simulink model "kurtosis_single_channel_subblocks"  (R2012b)
settings: Solver=ode45  StartTime=0.0  StopTime=3571  RelTol=1e-3
libraries: xbsIndex_r4 x454, xps_library x2, simulink_xsg_bridge x1
(part 2 of 4)

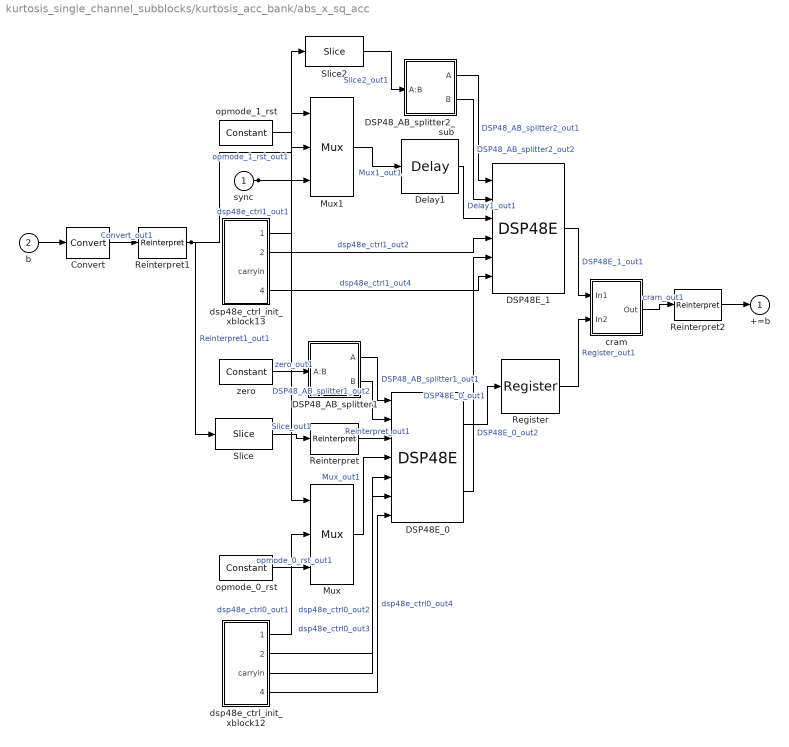
== system kurtosis_single_channel_subblocks/kurtosis_acc_bank/abs_x_sq_acc ==
  sync : Inport
  b : Inport  Port=2
  Convert : xbsIndex_r4/Convert  gui_display_data_type=Fixed-point  arith_type="Signed  (2's comp)"  n_bits=96  bin_pt=34  float_type=Single  exp_bits=8  fraction_bits=24  quantization=Truncate  overflow=Wrap  en=off  latency=0  dbl_ovrd=off  pipeline=off  block_type=convert
  DSP48E_0 : xbsIndex_r4/DSP48E  use_a=Direct from A Port  use_b=Direct from B Port  reset_preg=off  pattern_from_creg=on  pattern='000000000000'  mask_from_creg=on  pattern_mask='000000000000'  sel_rounding_mask=Select mask  use_op=off  use_creg=on  rst_all=off  en_all=off  use_pcin=off  use_carrycascin=off  use_multsignin=off  use_carryout=on  use_patterndetect=off  use_patternbdetect=off  use_overflow=off  use_underflow=off  use_acout=off  use_bcout=off  use_pcout=off  use_multsignout=off  use_carrycascout=off  pipeline_a=1  pipeline_b=1  pipeline_acout=1  pipeline_bcout=1  pipeline_c=on  pipeline_p=on  pipeline_mult=on  pipeline_opmode=on  pipeline_alumode=on  pipeline_carryin=on  pipeline_carryinsel=on  rst_a=off  rst_b=off  rst_c=off  rst_mult=off  rst_p=off  rst_carry_in=off  rst_alumode=off  rst_ctrl=off  en_a1=off  en_a2=off  en_b1=off  en_b2=off  en_c=off  en_mult=off  en_p=off  en_carry_in=off  en_alumode=off  en_multcarryin=off  en_ctrl=off  use_synth_model=off  addsub_mode=ONE48  xl_useadderonly=off  block_type=dsp48e
  DSP48E_1 : xbsIndex_r4/DSP48E  use_a=Direct from A Port  use_b=Direct from B Port  reset_preg=off  pattern_from_creg=on  pattern='000000000000'  mask_from_creg=on  pattern_mask='000000000000'  sel_rounding_mask=Select mask  use_op=off  use_creg=off  rst_all=off  en_all=off  use_pcin=off  use_carrycascin=off  use_multsignin=off  use_carryout=off  use_patterndetect=off  use_patternbdetect=off  use_overflow=off  use_underflow=off  use_acout=off  use_bcout=off  use_pcout=off  use_multsignout=off  use_carrycascout=off  pipeline_a=2  pipeline_b=2  pipeline_acout=1  pipeline_bcout=1  pipeline_c=on  pipeline_p=on  pipeline_mult=on  pipeline_opmode=on  pipeline_alumode=on  pipeline_carryin=off  pipeline_carryinsel=on  rst_a=off  rst_b=off  rst_c=off  rst_mult=off  rst_p=off  rst_carry_in=off  rst_alumode=off  rst_ctrl=off  en_a1=off  en_a2=off  en_b1=off  en_b2=off  en_c=off  en_mult=off  en_p=off  en_carry_in=off  en_alumode=off  en_multcarryin=off  en_ctrl=off  use_synth_model=off  addsub_mode=ONE48  xl_useadderonly=off  block_type=dsp48e
  DSP48_AB_splitter1 : Subsystem
  DSP48_AB_splitter2_sub : Subsystem
  Delay1 : xbsIndex_r4/Delay  rst=off  infoeditControl=Selection of Reset will increase slice count due to use of real FFs and instead of SRLs  en=off  latency=1  dbl_ovrd=off  reg_retiming=off  block_type=delay
  Mux : xbsIndex_r4/Mux  inputs=2  en=off  latency=0  precision=Full  arith_type=Unsigned  n_bits=16  bin_pt=14  quantization=Truncate  overflow=Wrap  dbl_ovrd=off  block_type=mux
  Mux1 : xbsIndex_r4/Mux  inputs=2  en=off  latency=0  precision=Full  arith_type=Unsigned  n_bits=16  bin_pt=14  quantization=Truncate  overflow=Wrap  dbl_ovrd=off  block_type=mux
  Register : xbsIndex_r4/Register  init=0  rst=off  en=off  dbl_ovrd=off  block_type=register
  Reinterpret : xbsIndex_r4/Reinterpret  force_arith_type=on  arith_type="Signed  (2's comp)"  force_bin_pt=on  bin_pt=0  block_type=reinterpret
  Reinterpret1 : xbsIndex_r4/Reinterpret  force_arith_type=on  arith_type="Signed  (2's comp)"  force_bin_pt=on  bin_pt=0  block_type=reinterpret
  Reinterpret2 : xbsIndex_r4/Reinterpret  force_arith_type=on  arith_type="Signed  (2's comp)"  force_bin_pt=on  bin_pt=34  block_type=reinterpret
  Slice : xbsIndex_r4/Slice  nbits=48  boolean_output=off  mode=Lower Bit Location + Width  bit1=0  base1=MSB of Input  bit0=0  base0=LSB of Input  dbl_ovrd=off  block_type=slice
  Slice2 : xbsIndex_r4/Slice  nbits=48  boolean_output=off  mode=Lower Bit Location + Width  bit1=0  base1=MSB of Input  bit0=48  base0=LSB of Input  dbl_ovrd=off  block_type=slice
  cram : Subsystem
  dsp48e_ctrl_init_xblock12 : Subsystem
  dsp48e_ctrl_init_xblock13 : Subsystem
  opmode_0_rst : xbsIndex_r4/Constant  const=12  gui_display_data_type=Fixed-point  arith_type=Unsigned  n_bits=7  bin_pt=0  preci_type=Single  exp_width=8  frac_width=24  explicit_period=on  period=1  equ=P=C  opselect=C  inp2=PCIN>>17  opr=+  inp1=P  carry=CIN  dbl_ovrd=off  block_type=constant
  opmode_1_rst : xbsIndex_r4/Constant  const=3  gui_display_data_type=Fixed-point  arith_type=Unsigned  n_bits=7  bin_pt=0  preci_type=Single  exp_width=8  frac_width=24  explicit_period=on  period=1  equ=P=C  opselect=C  inp2=PCIN>>17  opr=+  inp1=P  carry=CIN  dbl_ovrd=off  block_type=constant
  zero : xbsIndex_r4/Constant  const=0  gui_display_data_type=Fixed-point  arith_type=Signed (2's comp)  n_bits=48  bin_pt=0  preci_type=Single  exp_width=8  frac_width=24  explicit_period=on  period=1  equ=P=C  opselect=C  inp2=PCIN>>17  opr=+  inp1=P  carry=CIN  dbl_ovrd=off  block_type=constant
  +=b : Outport
  wires:
  sync/1 -> Mux1/1, Mux/1
  Reinterpret1/1 -> Slice2/1, Slice/1  "Reinterpret1_out1"
  dsp48e_ctrl_init_xblock13/4(carryinsel) -> DSP48E_1/6  "dsp48e_ctrl1_out4"
  dsp48e_ctrl_init_xblock13/2(alumode) -> DSP48E_1/4  "dsp48e_ctrl1_out2"
  dsp48e_ctrl_init_xblock13/1(opmode) -> Mux1/2  "dsp48e_ctrl1_out1"
  dsp48e_ctrl_init_xblock12/4(carryinsel) -> DSP48E_0/7  "dsp48e_ctrl0_out4"
  dsp48e_ctrl_init_xblock12/3(carryin) -> DSP48E_0/6  "dsp48e_ctrl0_out3"
  dsp48e_ctrl_init_xblock12/2(alumode) -> DSP48E_0/5  "dsp48e_ctrl0_out2"
  dsp48e_ctrl_init_xblock12/1(opmode) -> Mux/2  "dsp48e_ctrl0_out1"
  DSP48_AB_splitter2_sub/2(B) -> DSP48E_1/2  "DSP48_AB_splitter2_out2"
  DSP48_AB_splitter2_sub/1(A) -> DSP48E_1/1  "DSP48_AB_splitter2_out1"
  Slice2/1 -> DSP48_AB_splitter2_sub/1(A:B)  "Slice2_out1"
  zero/1 -> DSP48_AB_splitter1/1(A:B)  "zero_out1"
  opmode_1_rst/1 -> Mux1/3  "opmode_1_rst_out1"
  opmode_0_rst/1 -> Mux/3  "opmode_0_rst_out1"
  cram/1(Out) -> Reinterpret2/1  "cram_out1"
  Register/1 -> cram/2(In2)  "Register_out1"
  DSP48E_1/1 -> cram/1(In1)  "DSP48E_1_out1"
  Slice/1 -> Reinterpret/1  "Slice_out1"
  Reinterpret2/1 -> +=b/1
  Convert/1 -> Reinterpret1/1  "Convert_out1"
  Reinterpret/1 -> DSP48E_0/3  "Reinterpret_out1"
  DSP48E_0/1 -> Register/1  "DSP48E_0_out1"
  Mux1/1 -> Delay1/1  "Mux1_out1"
  Mux/1 -> DSP48E_0/4  "Mux_out1"
  Delay1/1 -> DSP48E_1/3  "Delay1_out1"
  DSP48_AB_splitter1/2(B) -> DSP48E_0/2  "DSP48_AB_splitter1_out2"
  DSP48_AB_splitter1/1(A) -> DSP48E_0/1  "DSP48_AB_splitter1_out1"
  DSP48E_0/2 -> DSP48E_1/5  "DSP48E_0_out2"
  b/1 -> Convert/1

== system kurtosis_single_channel_subblocks/kurtosis_acc_bank/acc_rst ==
  sync : Inport
  Constant5 : xbsIndex_r4/Constant  const=1023  gui_display_data_type=Fixed-point  arith_type=Unsigned  n_bits=11  bin_pt=0  preci_type=Single  exp_width=8  frac_width=24  explicit_period=on  period=1  equ=P=C  opselect=C  inp2=PCIN>>17  opr=+  inp1=P  carry=CIN  dbl_ovrd=off  block_type=constant
  Counter : xbsIndex_r4/Counter  cnt_type=Free Running  cnt_to=Inf  operation=Up  start_count=0  cnt_by_val=1  arith_type=Unsigned  n_bits=10  bin_pt=0  load_pin=off  rst=on  en=off  explicit_period=on  period=1  dbl_ovrd=off  use_behavioral_HDL=off  implementation=Fabric  block_type=counter
  Logical : xbsIndex_r4/Logical  logical_function=OR  inputs=2  en=off  latency=0  precision=Full  arith_type=Unsigned  n_bits=16  bin_pt=0  align_bp=on  dbl_ovrd=off  block_type=logical
  Relational : xbsIndex_r4/Relational  mode=a=b  en=off  latency=0  dbl_ovrd=off  block_type=relational
  acc_del : xbsIndex_r4/Delay  rst=off  infoeditControl=Selection of Reset will increase slice count due to use of real FFs and instead of SRLs  en=off  latency=2  dbl_ovrd=off  reg_retiming=off  block_type=delay
  sync_del : xbsIndex_r4/Delay  rst=off  infoeditControl=Selection of Reset will increase slice count due to use of real FFs and instead of SRLs  en=off  latency=1  dbl_ovrd=off  reg_retiming=off  block_type=delay
  acc_rst : Outport
  sync_out : Outport  Port=2
  wires:
  sync/1 -> Logical/2, Counter/1
  Relational/1 -> sync_del/1, acc_del/1  "Relational_out1"
  sync_del/1 -> Logical/1  "sync_del_out1"
  acc_del/1 -> sync_out/1
  Constant5/1 -> Relational/2  "Constant5_out1"
  Counter/1 -> Relational/1  "Counter_out1"
  Logical/1 -> acc_rst/1

== system kurtosis_single_channel_subblocks/kurtosis_acc_bank/x_acc ==
  sync : Inport
  x : Inport  Port=2
  c_to_ri : Subsystem
      settings: AttributesFormatString=55_51 r/i
  im_acc : Subsystem
  re_acc : Subsystem
  x_re_acc : Outport
  x_im_acc : Outport  Port=2
  wires:
  sync/1 -> im_acc/1(sync), re_acc/1(sync)
  im_acc/1(+=b) -> x_im_acc/1
  c_to_ri/2(im) -> im_acc/2(b)  "x_im"
  re_acc/1(+=b) -> x_re_acc/1
  c_to_ri/1(re) -> re_acc/2(b)  "x_re"
  x/1 -> c_to_ri/1(c)

== system kurtosis_single_channel_subblocks/kurtosis_acc_bank/x_cube_acc ==
  sync : Inport
  x : Inport  Port=2
  c_to_ri : Subsystem
  im_acc : Subsystem
  re_acc : Subsystem
  x_re_acc : Outport
  x_im_acc : Outport  Port=2
  wires:
  sync/1 -> im_acc/1(sync), re_acc/1(sync)
  im_acc/1(+=b) -> x_im_acc/1
  c_to_ri/2(im) -> im_acc/2(b)  "x_im"
  re_acc/1(+=b) -> x_re_acc/1
  c_to_ri/1(re) -> re_acc/2(b)  "x_re"
  x/1 -> c_to_ri/1(c)

== system kurtosis_single_channel_subblocks/kurtosis_acc_bank/x_sq_acc ==
  sync : Inport
  x : Inport  Port=2
  c_to_ri : Subsystem
  im_acc : Subsystem
  re_acc : Subsystem
  x_re_acc : Outport
  x_im_acc : Outport  Port=2
  wires:
  sync/1 -> im_acc/1(sync), re_acc/1(sync)
  im_acc/1(+=b) -> x_im_acc/1
  c_to_ri/2(im) -> im_acc/2(b)  "x_im"
  re_acc/1(+=b) -> x_re_acc/1
  c_to_ri/1(re) -> re_acc/2(b)  "x_re"
  x/1 -> c_to_ri/1(c)

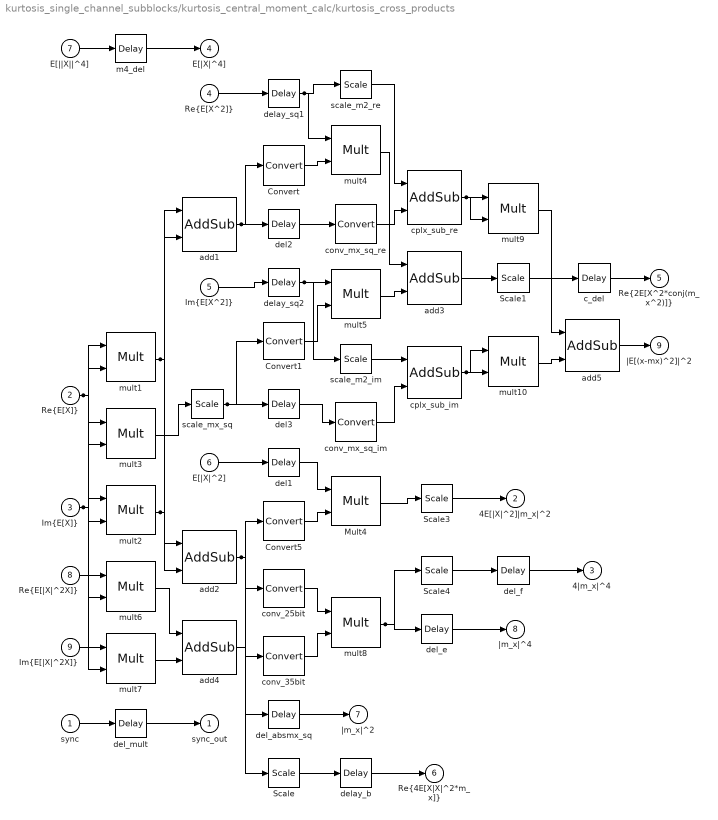
== system kurtosis_single_channel_subblocks/kurtosis_central_moment_calc/kurtosis_cross_products ==
  sync : Inport
  "Re{E[X]}" : Inport  Port=2
  "Im{E[X]}" : Inport  Port=3
  "Re{E[X^2]}" : Inport  Port=4
  "Im{E[X^2]}" : Inport  Port=5
  E[|X|^2] : Inport  Port=6
  E[||X||^4] : Inport  Port=7
  "Re{E[|X|^2X]}" : Inport  Port=8
  "Im{E[|X|^2X]}" : Inport  Port=9
  Convert : xbsIndex_r4/Convert  gui_display_data_type=Fixed-point  arith_type="Signed  (2's comp)"  n_bits=25  bin_pt=22  float_type=Single  exp_bits=8  fraction_bits=24  quantization="Round  (unbiased: +/- Inf)"  overflow=Saturate  en=off  latency=1  dbl_ovrd=off  pipeline=off  block_type=convert
  Convert1 : xbsIndex_r4/Convert  gui_display_data_type=Fixed-point  arith_type="Signed  (2's comp)"  n_bits=25  bin_pt=22  float_type=Single  exp_bits=8  fraction_bits=24  quantization="Round  (unbiased: +/- Inf)"  overflow=Saturate  en=off  latency=1  dbl_ovrd=off  pipeline=off  block_type=convert
  Convert5 : xbsIndex_r4/Convert  gui_display_data_type=Fixed-point  arith_type="Signed  (2's comp)"  n_bits=25  bin_pt=22  float_type=Single  exp_bits=8  fraction_bits=24  quantization="Round  (unbiased: +/- Inf)"  overflow=Saturate  en=off  latency=5  dbl_ovrd=off  pipeline=off  block_type=convert
  Mult4 : xbsIndex_r4/Mult  precision=Full  arith_type="Signed  (2's comp)"  n_bits=36  bin_pt=34  quantization=Truncate  overflow=Wrap  en=off  latency=5  dbl_ovrd=off  use_behavioral_HDL=off  opt=Speed  use_embedded=on  optimum_pipeline=off  pipeline=on  use_rpm=on  placement_style=Triangular  block_type=mult
  Scale : xbsIndex_r4/Scale  scale_factor=2  dbl_ovrd=off  block_type=scale
  Scale1 : xbsIndex_r4/Scale  scale_factor=1  dbl_ovrd=off  block_type=scale
  Scale3 : xbsIndex_r4/Scale  scale_factor=2  dbl_ovrd=off  block_type=scale
  Scale4 : xbsIndex_r4/Scale  scale_factor=2  dbl_ovrd=off  block_type=scale
  add1 : xbsIndex_r4/AddSub  mode=Subtraction  use_carryin=off  use_carryout=off  en=off  latency=2  precision=Full  arith_type="Signed  (2's comp)"  n_bits=36  bin_pt=34  quantization=Truncate  overflow=Wrap  dbl_ovrd=off  use_behavioral_HDL=off  hw_selection=Fabric  pipelined=off  block_type=addsub
  add2 : xbsIndex_r4/AddSub  mode=Addition  use_carryin=off  use_carryout=off  en=off  latency=2  precision=Full  arith_type="Signed  (2's comp)"  n_bits=36  bin_pt=34  quantization=Truncate  overflow=Wrap  dbl_ovrd=off  use_behavioral_HDL=off  hw_selection=Fabric  pipelined=off  block_type=addsub
  add3 : xbsIndex_r4/AddSub  mode=Addition  use_carryin=off  use_carryout=off  en=off  latency=2  precision=Full  arith_type="Signed  (2's comp)"  n_bits=36  bin_pt=34  quantization=Truncate  overflow=Wrap  dbl_ovrd=off  use_behavioral_HDL=off  hw_selection=Fabric  pipelined=off  block_type=addsub
  add4 : xbsIndex_r4/AddSub  mode=Addition  use_carryin=off  use_carryout=off  en=off  latency=2  precision=Full  arith_type="Signed  (2's comp)"  n_bits=36  bin_pt=34  quantization=Truncate  overflow=Wrap  dbl_ovrd=off  use_behavioral_HDL=off  hw_selection=Fabric  pipelined=off  block_type=addsub
  add5 : xbsIndex_r4/AddSub  mode=Addition  use_carryin=off  use_carryout=off  en=off  latency=3  precision=Full  arith_type="Signed  (2's comp)"  n_bits=36  bin_pt=34  quantization=Truncate  overflow=Wrap  dbl_ovrd=off  use_behavioral_HDL=off  hw_selection=Fabric  pipelined=off  block_type=addsub
  c_del : xbsIndex_r4/Delay  rst=off  infoeditControl=Selection of Reset will increase slice count due to use of real FFs and instead of SRLs  en=off  latency=4  dbl_ovrd=off  reg_retiming=off  block_type=delay
  conv_25bit : xbsIndex_r4/Convert  gui_display_data_type=Fixed-point  arith_type="Signed  (2's comp)"  n_bits=25  bin_pt=22  float_type=Single  exp_bits=8  fraction_bits=24  quantization="Round  (unbiased: +/- Inf)"  overflow=Saturate  en=off  latency=3  dbl_ovrd=off  pipeline=off  block_type=convert
  conv_35bit : xbsIndex_r4/Convert  gui_display_data_type=Fixed-point  arith_type="Signed  (2's comp)"  n_bits=35  bin_pt=32  float_type=Single  exp_bits=8  fraction_bits=24  quantization="Round  (unbiased: +/- Inf)"  overflow=Saturate  en=off  latency=3  dbl_ovrd=off  pipeline=off  block_type=convert
  conv_mx_sq_im : xbsIndex_r4/Convert  gui_display_data_type=Fixed-point  arith_type="Signed  (2's comp)"  n_bits=35  bin_pt=32  float_type=Single  exp_bits=8  fraction_bits=24  quantization="Round  (unbiased: +/- Inf)"  overflow=Saturate  en=off  latency=0  dbl_ovrd=off  pipeline=off  block_type=convert
  conv_mx_sq_re : xbsIndex_r4/Convert  gui_display_data_type=Fixed-point  arith_type="Signed  (2's comp)"  n_bits=35  bin_pt=32  float_type=Single  exp_bits=8  fraction_bits=24  quantization="Round  (unbiased: +/- Inf)"  overflow=Saturate  en=off  latency=0  dbl_ovrd=off  pipeline=off  block_type=convert
  cplx_sub_im : xbsIndex_r4/AddSub  mode=Subtraction  use_carryin=off  use_carryout=off  en=off  latency=2  precision=Full  arith_type="Signed  (2's comp)"  n_bits=36  bin_pt=34  quantization=Truncate  overflow=Wrap  dbl_ovrd=off  use_behavioral_HDL=off  hw_selection=Fabric  pipelined=off  block_type=addsub
  cplx_sub_re : xbsIndex_r4/AddSub  mode=Subtraction  use_carryin=off  use_carryout=off  en=off  latency=2  precision=Full  arith_type="Signed  (2's comp)"  n_bits=36  bin_pt=34  quantization=Truncate  overflow=Wrap  dbl_ovrd=off  use_behavioral_HDL=off  hw_selection=Fabric  pipelined=off  block_type=addsub
  del1 : xbsIndex_r4/Delay  rst=off  infoeditControl=Selection of Reset will increase slice count due to use of real FFs and instead of SRLs  en=off  latency=10  dbl_ovrd=off  reg_retiming=off  block_type=delay
  del2 : xbsIndex_r4/Delay  rst=off  infoeditControl=Selection of Reset will increase slice count due to use of real FFs and instead of SRLs  en=off  latency=1  dbl_ovrd=off  reg_retiming=off  block_type=delay
  del3 : xbsIndex_r4/Delay  rst=off  infoeditControl=Selection of Reset will increase slice count due to use of real FFs and instead of SRLs  en=off  latency=1  dbl_ovrd=off  reg_retiming=off  block_type=delay
  del_absmx_sq : xbsIndex_r4/Delay  rst=off  infoeditControl=Selection of Reset will increase slice count due to use of real FFs and instead of SRLs  en=off  latency=10  dbl_ovrd=off  reg_retiming=off  block_type=delay
  del_e : xbsIndex_r4/Delay  rst=off  infoeditControl=Selection of Reset will increase slice count due to use of real FFs and instead of SRLs  en=off  latency=2  dbl_ovrd=off  reg_retiming=off  block_type=delay
  del_f : xbsIndex_r4/Delay  rst=off  infoeditControl=Selection of Reset will increase slice count due to use of real FFs and instead of SRLs  en=off  latency=2  dbl_ovrd=off  reg_retiming=off  block_type=delay
  del_mult : xbsIndex_r4/Delay  rst=off  infoeditControl=Selection of Reset will increase slice count due to use of real FFs and instead of SRLs  en=off  latency=15  dbl_ovrd=off  reg_retiming=off  block_type=delay
  delay_b : xbsIndex_r4/Delay  rst=off  infoeditControl=Selection of Reset will increase slice count due to use of real FFs and instead of SRLs  en=off  latency=7  dbl_ovrd=off  reg_retiming=off  block_type=delay
  delay_sq1 : xbsIndex_r4/Delay  rst=off  infoeditControl=Selection of Reset will increase slice count due to use of real FFs and instead of SRLs  en=off  latency=6  dbl_ovrd=off  reg_retiming=off  block_type=delay
  delay_sq2 : xbsIndex_r4/Delay  rst=off  infoeditControl=Selection of Reset will increase slice count due to use of real FFs and instead of SRLs  en=off  latency=6  dbl_ovrd=off  reg_retiming=off  block_type=delay
  m4_del : xbsIndex_r4/Delay  rst=off  infoeditControl=Selection of Reset will increase slice count due to use of real FFs and instead of SRLs  en=off  latency=15  dbl_ovrd=off  reg_retiming=off  block_type=delay
  mult{1..2,4..5} (4 alike) : xbsIndex_r4/Mult  precision=Full  arith_type="Signed  (2's comp)"  n_bits=36  bin_pt=34  quantization=Truncate  overflow=Wrap  en=off  latency=3  dbl_ovrd=off  use_behavioral_HDL=off  opt=Speed  use_embedded=on  optimum_pipeline=off  pipeline=on  use_rpm=on  placement_style=Triangular  block_type=mult
  mult10 : xbsIndex_r4/Mult  precision=Full  arith_type="Signed  (2's comp)"  n_bits=36  bin_pt=34  quantization=Truncate  overflow=Wrap  en=off  latency=4  dbl_ovrd=off  use_behavioral_HDL=off  opt=Speed  use_embedded=on  optimum_pipeline=off  pipeline=on  use_rpm=on  placement_style=Triangular  block_type=mult
  mult3 : xbsIndex_r4/Mult  precision=Full  arith_type="Signed  (2's comp)"  n_bits=36  bin_pt=34  quantization=Truncate  overflow=Wrap  en=off  latency=5  dbl_ovrd=off  use_behavioral_HDL=off  opt=Speed  use_embedded=on  optimum_pipeline=off  pipeline=on  use_rpm=on  placement_style=Triangular  block_type=mult
  mult6 : xbsIndex_r4/Mult  precision=Full  arith_type="Signed  (2's comp)"  n_bits=36  bin_pt=34  quantization=Truncate  overflow=Wrap  en=off  latency=6  dbl_ovrd=off  use_behavioral_HDL=off  opt=Speed  use_embedded=on  optimum_pipeline=off  pipeline=on  use_rpm=on  placement_style=Triangular  block_type=mult
  mult7 : xbsIndex_r4/Mult  precision=Full  arith_type="Signed  (2's comp)"  n_bits=36  bin_pt=34  quantization=Truncate  overflow=Wrap  en=off  latency=6  dbl_ovrd=off  use_behavioral_HDL=off  opt=Speed  use_embedded=on  optimum_pipeline=off  pipeline=on  use_rpm=on  placement_style=Triangular  block_type=mult
  mult8 : xbsIndex_r4/Mult  precision=Full  arith_type="Signed  (2's comp)"  n_bits=36  bin_pt=34  quantization=Truncate  overflow=Wrap  en=off  latency=5  dbl_ovrd=off  use_behavioral_HDL=off  opt=Speed  use_embedded=on  optimum_pipeline=off  pipeline=on  use_rpm=on  placement_style=Triangular  block_type=mult
  mult9 : xbsIndex_r4/Mult  precision=Full  arith_type="Signed  (2's comp)"  n_bits=36  bin_pt=34  quantization=Truncate  overflow=Wrap  en=off  latency=4  dbl_ovrd=off  use_behavioral_HDL=off  opt=Speed  use_embedded=on  optimum_pipeline=off  pipeline=on  use_rpm=on  placement_style=Triangular  block_type=mult
  scale_m2_im : xbsIndex_r4/Scale  scale_factor=-10  dbl_ovrd=off  block_type=scale
  scale_m2_re : xbsIndex_r4/Scale  scale_factor=-10  dbl_ovrd=off  block_type=scale
  scale_mx_sq : xbsIndex_r4/Scale  scale_factor=1  dbl_ovrd=off  block_type=scale
  sync_out : Outport
  4E[|X|^2]|m_x|^2 : Outport  Port=2
  4|m_x|^4 : Outport  Port=3
  E[|X|^4] : Outport  Port=4
  "Re{2E[X^2*conj(m_x^2)]}" : Outport  Port=5
  "Re{4E[X|X|^2*m_x]}" : Outport  Port=6
  |m_x|^2 : Outport  Port=7
  |m_x|^4 : Outport  Port=8
  |E[(x-mx)^2]|^2 : Outport  Port=9
  wires:
  "Re{E[X]}"/1 -> mult6/2, mult3/1, mult1/2, mult1/1
  "Im{E[X]}"/1 -> mult7/2, mult3/2, mult2/2, mult2/1
  mult1/1 -> add2/1, add1/1
  mult2/1 -> add2/2, add1/2
  add1/1 -> del2/1, Convert/1
  scale_mx_sq/1 -> del3/1, Convert1/1
  delay_sq1/1 -> scale_m2_re/1, mult4/1
  delay_sq2/1 -> scale_m2_im/1, mult5/1
  add2/1 -> del_absmx_sq/1, Convert5/1, conv_35bit/1, conv_25bit/1
  mult8/1 -> Scale4/1, del_e/1
  cplx_sub_re/1 -> mult9/2, mult9/1
  cplx_sub_im/1 -> mult10/2, mult10/1
  del_absmx_sq/1 -> |m_x|^2/1
  add5/1 -> |E[(x-mx)^2]|^2/1
  del_f/1 -> 4|m_x|^4/1
  del_e/1 -> |m_x|^4/1
  Scale3/1 -> 4E[|X|^2]|m_x|^2/1
  c_del/1 -> "Re{2E[X^2*conj(m_x^2)]}"/1
  delay_b/1 -> "Re{4E[X|X|^2*m_x]}"/1
  m4_del/1 -> E[|X|^4]/1
  E[||X||^4]/1 -> m4_del/1
  del_mult/1 -> sync_out/1
  sync/1 -> del_mult/1
  mult10/1 -> add5/2
  mult9/1 -> add5/1
  conv_mx_sq_im/1 -> cplx_sub_im/2
  scale_m2_im/1 -> cplx_sub_im/1
  conv_mx_sq_re/1 -> cplx_sub_re/2
  scale_m2_re/1 -> cplx_sub_re/1
  del3/1 -> conv_mx_sq_im/1
  del2/1 -> conv_mx_sq_re/1
  Scale4/1 -> del_f/1
  Mult4/1 -> Scale3/1
  Convert5/1 -> Mult4/2
  del1/1 -> Mult4/1
  E[|X|^2]/1 -> del1/1
  Scale1/1 -> c_del/1
  add3/1 -> Scale1/1
  Scale/1 -> delay_b/1
  add4/1 -> Scale/1
  conv_35bit/1 -> mult8/2
  conv_25bit/1 -> mult8/1
  mult7/1 -> add4/2
  mult6/1 -> add4/1
  "Im{E[|X|^2X]}"/1 -> mult7/1
  "Re{E[|X|^2X]}"/1 -> mult6/1
  mult5/1 -> add3/2
  mult4/1 -> add3/1
  Convert1/1 -> mult5/2
  Convert/1 -> mult4/2
  "Im{E[X^2]}"/1 -> delay_sq2/1
  "Re{E[X^2]}"/1 -> delay_sq1/1
  mult3/1 -> scale_mx_sq/1

== system kurtosis_single_channel_subblocks/kurtosis_central_moment_calc/kurtosis_den ==
  E[|X|^2] : Inport
  |m_x|^2 : Inport  Port=2
  Sub : xbsIndex_r4/AddSub  mode=Subtraction  use_carryin=off  use_carryout=off  en=off  latency=4  precision=Full  arith_type="Signed  (2's comp)"  n_bits=36  bin_pt=34  quantization=Truncate  overflow=Wrap  dbl_ovrd=off  use_behavioral_HDL=off  hw_selection=Fabric  pipelined=off  block_type=addsub
  conv : xbsIndex_r4/Convert  gui_display_data_type=Fixed-point  arith_type="Signed  (2's comp)"  n_bits=64  bin_pt=56  float_type=Single  exp_bits=8  fraction_bits=24  quantization="Round  (unbiased: +/- Inf)"  overflow=Saturate  en=off  latency=1  dbl_ovrd=off  pipeline=off  block_type=convert
  scale : xbsIndex_r4/Scale  scale_factor=-10  dbl_ovrd=off  block_type=scale
  square : xbsIndex_r4/Mult  precision=Full  arith_type="Signed  (2's comp)"  n_bits=36  bin_pt=34  quantization=Truncate  overflow=Wrap  en=off  latency=5  dbl_ovrd=off  use_behavioral_HDL=off  opt=Speed  use_embedded=on  optimum_pipeline=off  pipeline=on  use_rpm=on  placement_style=Triangular  block_type=mult
  square_conv_25bit : xbsIndex_r4/Convert  gui_display_data_type=Fixed-point  arith_type="Signed  (2's comp)"  n_bits=25  bin_pt=21  float_type=Single  exp_bits=8  fraction_bits=24  quantization="Round  (unbiased: +/- Inf)"  overflow=Saturate  en=off  latency=3  dbl_ovrd=off  pipeline=off  block_type=convert
  square_conv_35bit : xbsIndex_r4/Convert  gui_display_data_type=Fixed-point  arith_type="Signed  (2's comp)"  n_bits=35  bin_pt=31  float_type=Single  exp_bits=8  fraction_bits=24  quantization="Round  (unbiased: +/- Inf)"  overflow=Saturate  en=off  latency=3  dbl_ovrd=off  pipeline=off  block_type=convert
  E[|X-m_x|^2]^2 : Outport
  wires:
  Sub/1 -> square_conv_25bit/1, square_conv_35bit/1
  conv/1 -> E[|X-m_x|^2]^2/1
  square/1 -> conv/1
  square_conv_25bit/1 -> square/2
  square_conv_35bit/1 -> square/1
  |m_x|^2/1 -> Sub/2
  scale/1 -> Sub/1
  E[|X|^2]/1 -> scale/1

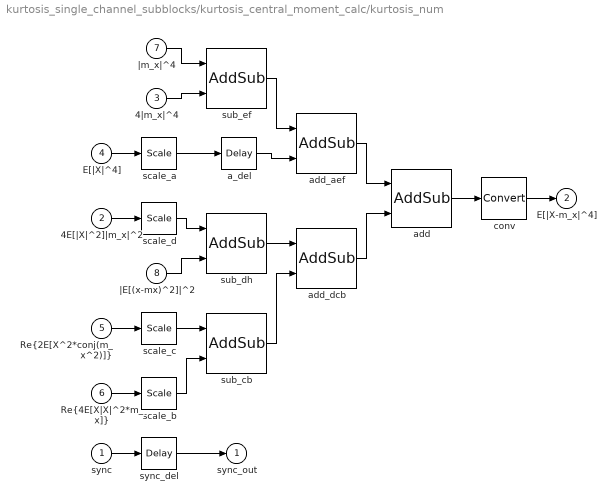
== system kurtosis_single_channel_subblocks/kurtosis_central_moment_calc/kurtosis_num ==
  sync : Inport
  4E[|X|^2]|m_x|^2 : Inport  Port=2
  4|m_x|^4 : Inport  Port=3
  E[|X|^4] : Inport  Port=4
  "Re{2E[X^2*conj(m_x^2)]}" : Inport  Port=5
  "Re{4E[X|X|^2*m_x]}" : Inport  Port=6
  |m_x|^4 : Inport  Port=7
  |E[(x-mx)^2]|^2 : Inport  Port=8
  a_del : xbsIndex_r4/Delay  rst=off  infoeditControl=Selection of Reset will increase slice count due to use of real FFs and instead of SRLs  en=off  latency=4  dbl_ovrd=off  reg_retiming=off  block_type=delay
  add : xbsIndex_r4/AddSub  mode=Addition  use_carryin=off  use_carryout=off  en=off  latency=4  precision=Full  arith_type="Signed  (2's comp)"  n_bits=36  bin_pt=34  quantization=Truncate  overflow=Wrap  dbl_ovrd=off  use_behavioral_HDL=off  hw_selection=Fabric  pipelined=off  block_type=addsub
  add_aef : xbsIndex_r4/AddSub  mode=Addition  use_carryin=off  use_carryout=off  en=off  latency=4  precision=Full  arith_type="Signed  (2's comp)"  n_bits=36  bin_pt=34  quantization=Truncate  overflow=Wrap  dbl_ovrd=off  use_behavioral_HDL=off  hw_selection=Fabric  pipelined=off  block_type=addsub
  add_dcb : xbsIndex_r4/AddSub  mode=Addition  use_carryin=off  use_carryout=off  en=off  latency=4  precision=Full  arith_type="Signed  (2's comp)"  n_bits=36  bin_pt=34  quantization=Truncate  overflow=Wrap  dbl_ovrd=off  use_behavioral_HDL=off  hw_selection=Fabric  pipelined=off  block_type=addsub
  conv : xbsIndex_r4/Convert  gui_display_data_type=Fixed-point  arith_type="Signed  (2's comp)"  n_bits=96  bin_pt=84  float_type=Single  exp_bits=8  fraction_bits=24  quantization="Round  (unbiased: +/- Inf)"  overflow=Saturate  en=off  latency=1  dbl_ovrd=off  pipeline=off  block_type=convert
  scale_a : xbsIndex_r4/Scale  scale_factor=-10  dbl_ovrd=off  block_type=scale
  scale_b : xbsIndex_r4/Scale  scale_factor=-10  dbl_ovrd=off  block_type=scale
  scale_c : xbsIndex_r4/Scale  scale_factor=-10  dbl_ovrd=off  block_type=scale
  scale_d : xbsIndex_r4/Scale  scale_factor=-10  dbl_ovrd=off  block_type=scale
  sub_cb : xbsIndex_r4/AddSub  mode=Subtraction  use_carryin=off  use_carryout=off  en=off  latency=4  precision=Full  arith_type="Signed  (2's comp)"  n_bits=36  bin_pt=34  quantization=Truncate  overflow=Wrap  dbl_ovrd=off  use_behavioral_HDL=off  hw_selection=Fabric  pipelined=off  block_type=addsub
  sub_dh : xbsIndex_r4/AddSub  mode=Subtraction  use_carryin=off  use_carryout=off  en=off  latency=4  precision=Full  arith_type="Signed  (2's comp)"  n_bits=36  bin_pt=34  quantization=Truncate  overflow=Wrap  dbl_ovrd=off  use_behavioral_HDL=off  hw_selection=Fabric  pipelined=off  block_type=addsub
  sub_ef : xbsIndex_r4/AddSub  mode=Subtraction  use_carryin=off  use_carryout=off  en=off  latency=4  precision=Full  arith_type="Signed  (2's comp)"  n_bits=36  bin_pt=34  quantization=Truncate  overflow=Wrap  dbl_ovrd=off  use_behavioral_HDL=off  hw_selection=Fabric  pipelined=off  block_type=addsub
  sync_del : xbsIndex_r4/Delay  rst=off  infoeditControl=Selection of Reset will increase slice count due to use of real FFs and instead of SRLs  en=off  latency=13  dbl_ovrd=off  reg_retiming=off  block_type=delay
  sync_out : Outport
  E[|X-m_x|^4] : Outport  Port=2
  wires:
  sync_del/1 -> sync_out/1
  conv/1 -> E[|X-m_x|^4]/1
  add/1 -> conv/1
  add_dcb/1 -> add/2
  add_aef/1 -> add/1
  sub_cb/1 -> add_dcb/2
  sub_dh/1 -> add_dcb/1
  a_del/1 -> add_aef/2
  sub_ef/1 -> add_aef/1
  scale_a/1 -> a_del/1
  |E[(x-mx)^2]|^2/1 -> sub_dh/2
  scale_d/1 -> sub_dh/1
  scale_b/1 -> sub_cb/2
  scale_c/1 -> sub_cb/1
  4|m_x|^4/1 -> sub_ef/2
  |m_x|^4/1 -> sub_ef/1
  4E[|X|^2]|m_x|^2/1 -> scale_d/1
  "Re{2E[X^2*conj(m_x^2)]}"/1 -> scale_c/1
  "Re{4E[X|X|^2*m_x]}"/1 -> scale_b/1
  E[|X|^4]/1 -> scale_a/1
  sync/1 -> sync_del/1

== system kurtosis_single_channel_subblocks/kurtosis_origin_moments/abs_x_sq ==
  c : Inport
  c_to_ri : Subsystem
  imag_square : xbsIndex_r4/Mult  precision=Full  arith_type="Signed  (2's comp)"  n_bits=16  bin_pt=14  quantization=Truncate  overflow=Wrap  en=off  latency=3  dbl_ovrd=off  use_behavioral_HDL=off  opt=Speed  use_embedded=on  optimum_pipeline=off  pipeline=on  use_rpm=on  placement_style=Rectangular shape  block_type=mult
  power_adder : xbsIndex_r4/AddSub  mode=Addition  use_carryin=off  use_carryout=off  en=off  latency=2  precision=Full  arith_type=Unsigned  n_bits=16  bin_pt=14  quantization=Truncate  overflow=Wrap  dbl_ovrd=off  use_behavioral_HDL=on  hw_selection=Fabric  pipelined=off  use_rpm=on  block_type=addsub
  real_square : xbsIndex_r4/Mult  precision=Full  arith_type="Signed  (2's comp)"  n_bits=16  bin_pt=14  quantization=Truncate  overflow=Wrap  en=off  latency=3  dbl_ovrd=off  use_behavioral_HDL=off  opt=Speed  use_embedded=on  optimum_pipeline=off  pipeline=on  use_rpm=on  placement_style=Triangular  block_type=mult
  power : Outport
  wires:
  c_to_ri/2(im) -> imag_square/2, imag_square/1
  c_to_ri/1(re) -> real_square/2, real_square/1
  real_square/1 -> power_adder/1
  power_adder/1 -> power/1
  imag_square/1 -> power_adder/2
  c/1 -> c_to_ri/1(c)

== system kurtosis_single_channel_subblocks/kurtosis_origin_moments/c_to_ri_xin ==
  c : Inport
  force_im : xbsIndex_r4/Reinterpret  force_arith_type=on  arith_type="Signed  (2's comp)"  force_bin_pt=on  bin_pt=17  block_type=reinterpret
  force_re : xbsIndex_r4/Reinterpret  force_arith_type=on  arith_type="Signed  (2's comp)"  force_bin_pt=on  bin_pt=17  block_type=reinterpret
  slice_im : xbsIndex_r4/Slice  nbits=18  boolean_output=off  mode=Lower Bit Location + Width  bit1=0  base1=MSB of Input  bit0=0  base0=LSB of Input  dbl_ovrd=off  block_type=slice
  slice_re : xbsIndex_r4/Slice  nbits=18  boolean_output=off  mode=Upper Bit Location + Width  bit1=0  base1=MSB of Input  bit0=0  base0=LSB of Input  dbl_ovrd=off  block_type=slice
  re : Outport
  im : Outport  Port=2
  wires:
  c/1 -> slice_im/1, slice_re/1
  force_im/1 -> im/1
  slice_im/1 -> force_im/1
  force_re/1 -> re/1
  slice_re/1 -> force_re/1

== system kurtosis_single_channel_subblocks/kurtosis_origin_moments/cplx_sq ==
  a : Inport
  b : Inport  Port=2
  AddSub : xbsIndex_r4/AddSub  mode=Subtraction  use_carryin=off  use_carryout=off  en=off  latency=2  precision=Full  arith_type=Unsigned  n_bits=16  bin_pt=14  quantization=Truncate  overflow=Wrap  dbl_ovrd=off  use_behavioral_HDL=on  hw_selection=Fabric  pipelined=off  block_type=addsub
  AddSub1 : xbsIndex_r4/AddSub  mode=Addition  use_carryin=off  use_carryout=off  en=off  latency=2  precision=Full  arith_type=Unsigned  n_bits=16  bin_pt=14  quantization=Truncate  overflow=Wrap  dbl_ovrd=off  use_behavioral_HDL=on  hw_selection=Fabric  pipelined=off  block_type=addsub
  a_input_c_to_ri : Subsystem
  b_input_c_to_ri : Subsystem
  c_output_ri_to_c : Subsystem
  convert0 : xbsIndex_r4/Convert  gui_display_data_type=Fixed-point  arith_type="Signed  (2's comp)"  n_bits=37  bin_pt=34  float_type=Single  exp_bits=8  fraction_bits=24  quantization=Truncate  overflow=Wrap  en=off  latency=1  dbl_ovrd=off  pipeline=on  block_type=convert
  convert1 : xbsIndex_r4/Convert  gui_display_data_type=Fixed-point  arith_type="Signed  (2's comp)"  n_bits=37  bin_pt=34  float_type=Single  exp_bits=8  fraction_bits=24  quantization=Truncate  overflow=Wrap  en=off  latency=1  dbl_ovrd=off  pipeline=on  block_type=convert
  mults : Subsystem
  c : Outport
  wires:
  a_input_c_to_ri/1(re) -> mults/7(a4), mults/1(a1)  "a_re"
  b_input_c_to_ri/1(re) -> mults/6(b3), mults/2(b1)  "b_re"
  a_input_c_to_ri/2(im) -> mults/5(a3), mults/3(a2)  "a_im"
  b_input_c_to_ri/2(im) -> mults/8(b4), mults/4(b2)  "b_im"
  convert1/1 -> c_output_ri_to_c/2(im)  "c_im"
  AddSub1/1 -> convert1/1
  convert0/1 -> c_output_ri_to_c/1(re)  "c_re"
  AddSub/1 -> convert0/1
  mults/4(c4) -> AddSub1/2
  mults/3(c3) -> AddSub1/1
  mults/2(c2) -> AddSub/2
  mults/1(c1) -> AddSub/1
  c_output_ri_to_c/1(c) -> c/1
  b/1 -> b_input_c_to_ri/1(c)
  a/1 -> a_input_c_to_ri/1(c)

== system kurtosis_single_channel_subblocks/kurtosis_origin_moments/ri_to_c_x_3rd ==
  re : Inport
  im : Inport  Port=2
  concat : xbsIndex_r4/Concat  num_inputs=2  dbl_ovrd=off  block_type=concat
  force_im : xbsIndex_r4/Reinterpret  force_arith_type=on  arith_type=Unsigned  force_bin_pt=on  bin_pt=0  block_type=reinterpret
  force_re : xbsIndex_r4/Reinterpret  force_arith_type=on  arith_type=Unsigned  force_bin_pt=on  bin_pt=0  block_type=reinterpret
  c : Outport
  wires:
  force_re/1 -> concat/1
  re/1 -> force_re/1
  force_im/1 -> concat/2
  im/1 -> force_im/1
  concat/1 -> c/1

== system kurtosis_single_channel_subblocks/to_workspace_complex/c_to_ri ==
  c : Inport
  force_im : xbsIndex_r4/Reinterpret  force_arith_type=on  arith_type="Signed  (2's comp)"  force_bin_pt=on  bin_pt=17  block_type=reinterpret
  force_re : xbsIndex_r4/Reinterpret  force_arith_type=on  arith_type="Signed  (2's comp)"  force_bin_pt=on  bin_pt=17  block_type=reinterpret
  slice_im : xbsIndex_r4/Slice  nbits=18  boolean_output=off  mode=Lower Bit Location + Width  bit1=0  base1=MSB of Input  bit0=0  base0=LSB of Input  dbl_ovrd=off  block_type=slice
  slice_re : xbsIndex_r4/Slice  nbits=18  boolean_output=off  mode=Upper Bit Location + Width  bit1=0  base1=MSB of Input  bit0=0  base0=LSB of Input  dbl_ovrd=off  block_type=slice
  re : Outport
  im : Outport  Port=2
  wires:
  c/1 -> slice_im/1, slice_re/1
  force_im/1 -> im/1
  slice_im/1 -> force_im/1
  force_re/1 -> re/1
  slice_re/1 -> force_re/1

== system kurtosis_single_channel_subblocks/kurtosis_acc_bank/abs_x_4th_acc/DSP48_AB_splitter1 ==
  A:B : Inport
  Reinterpret1 : xbsIndex_r4/Reinterpret  force_arith_type=on  arith_type="Signed  (2's comp)"  force_bin_pt=on  bin_pt=0  block_type=reinterpret
  Reinterpret2 : xbsIndex_r4/Reinterpret  force_arith_type=on  arith_type="Signed  (2's comp)"  force_bin_pt=on  bin_pt=0  block_type=reinterpret
  Slice1 : xbsIndex_r4/Slice  nbits=30  boolean_output=off  mode=Lower Bit Location + Width  bit1=0  base1=MSB of Input  bit0=18  base0=LSB of Input  dbl_ovrd=off  block_type=slice
  Slice3 : xbsIndex_r4/Slice  nbits=18  boolean_output=off  mode=Lower Bit Location + Width  bit1=0  base1=MSB of Input  bit0=0  base0=LSB of Input  dbl_ovrd=off  block_type=slice
  A : Outport
  B : Outport  Port=2
  wires:
  A:B/1 -> Slice3/1, Slice1/1
  Slice3/1 -> Reinterpret1/1  "Slice3_out1"
  Slice1/1 -> Reinterpret2/1  "Slice1_out1"
  Reinterpret2/1 -> A/1
  Reinterpret1/1 -> B/1

== system kurtosis_single_channel_subblocks/kurtosis_acc_bank/abs_x_4th_acc/DSP48_AB_splitter2_sub ==
  A:B : Inport
  Reinterpret1 : xbsIndex_r4/Reinterpret  force_arith_type=on  arith_type="Signed  (2's comp)"  force_bin_pt=on  bin_pt=0  block_type=reinterpret
  Reinterpret2 : xbsIndex_r4/Reinterpret  force_arith_type=on  arith_type="Signed  (2's comp)"  force_bin_pt=on  bin_pt=0  block_type=reinterpret
  Slice1 : xbsIndex_r4/Slice  nbits=30  boolean_output=off  mode=Lower Bit Location + Width  bit1=0  base1=MSB of Input  bit0=18  base0=LSB of Input  dbl_ovrd=off  block_type=slice
  Slice3 : xbsIndex_r4/Slice  nbits=18  boolean_output=off  mode=Lower Bit Location + Width  bit1=0  base1=MSB of Input  bit0=0  base0=LSB of Input  dbl_ovrd=off  block_type=slice
  A : Outport
  B : Outport  Port=2
  wires:
  A:B/1 -> Slice3/1, Slice1/1
  Slice3/1 -> Reinterpret1/1  "Slice3_out1"
  Slice1/1 -> Reinterpret2/1  "Slice1_out1"
  Reinterpret2/1 -> A/1
  Reinterpret1/1 -> B/1

== system kurtosis_single_channel_subblocks/kurtosis_acc_bank/abs_x_4th_acc/cram ==
  In1 : Inport
  In2 : Inport  Port=2
  Concat : xbsIndex_r4/Concat  num_inputs=2  dbl_ovrd=off  block_type=concat
  Reinterp1 : xbsIndex_r4/Reinterpret  force_arith_type=on  arith_type=Unsigned  force_bin_pt=on  bin_pt=0  block_type=reinterpret
  Reinterp2 : xbsIndex_r4/Reinterpret  force_arith_type=on  arith_type=Unsigned  force_bin_pt=on  bin_pt=0  block_type=reinterpret
  Out : Outport
  wires:
  Concat/1 -> Out/1
  Reinterp2/1 -> Concat/2
  Reinterp1/1 -> Concat/1
  In2/1 -> Reinterp2/1
  In1/1 -> Reinterp1/1

== system kurtosis_single_channel_subblocks/kurtosis_acc_bank/abs_x_4th_acc/dsp48e_ctrl_init_xblock14 ==
  alumode0 : xbsIndex_r4/Constant  const=0  gui_display_data_type=Fixed-point  arith_type=Unsigned  n_bits=4  bin_pt=0  preci_type=Single  exp_width=8  frac_width=24  explicit_period=off  period=1  equ=P=C  opselect=C  inp2=PCIN>>17  opr=+  inp1=P  carry=CIN  dbl_ovrd=off  block_type=constant
  carryin0 : xbsIndex_r4/Constant  const=0  gui_display_data_type=Fixed-point  arith_type=Unsigned  n_bits=1  bin_pt=0  preci_type=Single  exp_width=8  frac_width=24  explicit_period=off  period=1  equ=P=C  opselect=C  inp2=PCIN>>17  opr=+  inp1=P  carry=CIN  dbl_ovrd=off  block_type=constant
  carryinsel0 : xbsIndex_r4/Constant  const=0  gui_display_data_type=Fixed-point  arith_type=Unsigned  n_bits=3  bin_pt=0  preci_type=Single  exp_width=8  frac_width=24  explicit_period=off  period=1  equ=P=C  opselect=C  inp2=PCIN>>17  opr=+  inp1=P  carry=CIN  dbl_ovrd=off  block_type=constant
  opmode0 : xbsIndex_r4/Constant  const=44  gui_display_data_type=Fixed-point  arith_type=Unsigned  n_bits=7  bin_pt=0  preci_type=Single  exp_width=8  frac_width=24  explicit_period=off  period=1  equ=P=C  opselect=C  inp2=PCIN>>17  opr=+  inp1=P  carry=CIN  dbl_ovrd=off  block_type=constant
  opmode : Outport
  alumode : Outport  Port=2
  carryin : Outport  Port=3
  carryinsel : Outport  Port=4
  wires:
  opmode0/1 -> opmode/1
  carryinsel0/1 -> carryinsel/1
  carryin0/1 -> carryin/1
  alumode0/1 -> alumode/1

== system kurtosis_single_channel_subblocks/kurtosis_acc_bank/abs_x_4th_acc/dsp48e_ctrl_init_xblock15 ==
  alumode0 : xbsIndex_r4/Constant  const=0  gui_display_data_type=Fixed-point  arith_type=Unsigned  n_bits=4  bin_pt=0  preci_type=Single  exp_width=8  frac_width=24  explicit_period=off  period=1  equ=P=C  opselect=C  inp2=PCIN>>17  opr=+  inp1=P  carry=CIN  dbl_ovrd=off  block_type=constant
  carryin0 : xbsIndex_r4/Constant  const=0  gui_display_data_type=Fixed-point  arith_type=Unsigned  n_bits=1  bin_pt=0  preci_type=Single  exp_width=8  frac_width=24  explicit_period=off  period=1  equ=P=C  opselect=C  inp2=PCIN>>17  opr=+  inp1=P  carry=CIN  dbl_ovrd=off  block_type=constant
  carryinsel0 : xbsIndex_r4/Constant  const=0  gui_display_data_type=Fixed-point  arith_type=Unsigned  n_bits=3  bin_pt=0  preci_type=Single  exp_width=8  frac_width=24  explicit_period=off  period=1  equ=P=C  opselect=C  inp2=PCIN>>17  opr=+  inp1=P  carry=CIN  dbl_ovrd=off  block_type=constant
  opmode0 : xbsIndex_r4/Constant  const=35  gui_display_data_type=Fixed-point  arith_type=Unsigned  n_bits=7  bin_pt=0  preci_type=Single  exp_width=8  frac_width=24  explicit_period=off  period=1  equ=P=C  opselect=C  inp2=PCIN>>17  opr=+  inp1=P  carry=CIN  dbl_ovrd=off  block_type=constant
  opmode : Outport
  alumode : Outport  Port=2
  carryin : Outport  Port=3
  carryinsel : Outport  Port=4
  wires:
  opmode0/1 -> opmode/1
  carryinsel0/1 -> carryinsel/1
  carryin0/1 -> carryin/1
  alumode0/1 -> alumode/1

== system kurtosis_single_channel_subblocks/kurtosis_acc_bank/abs_x_sq_acc/DSP48_AB_splitter1 ==
  A:B : Inport
  Reinterpret1 : xbsIndex_r4/Reinterpret  force_arith_type=on  arith_type="Signed  (2's comp)"  force_bin_pt=on  bin_pt=0  block_type=reinterpret
  Reinterpret2 : xbsIndex_r4/Reinterpret  force_arith_type=on  arith_type="Signed  (2's comp)"  force_bin_pt=on  bin_pt=0  block_type=reinterpret
  Slice1 : xbsIndex_r4/Slice  nbits=30  boolean_output=off  mode=Lower Bit Location + Width  bit1=0  base1=MSB of Input  bit0=18  base0=LSB of Input  dbl_ovrd=off  block_type=slice
  Slice3 : xbsIndex_r4/Slice  nbits=18  boolean_output=off  mode=Lower Bit Location + Width  bit1=0  base1=MSB of Input  bit0=0  base0=LSB of Input  dbl_ovrd=off  block_type=slice
  A : Outport
  B : Outport  Port=2
  wires:
  A:B/1 -> Slice3/1, Slice1/1
  Slice3/1 -> Reinterpret1/1  "Slice3_out1"
  Slice1/1 -> Reinterpret2/1  "Slice1_out1"
  Reinterpret2/1 -> A/1
  Reinterpret1/1 -> B/1

== system kurtosis_single_channel_subblocks/kurtosis_acc_bank/abs_x_sq_acc/DSP48_AB_splitter2_sub ==
  A:B : Inport
  Reinterpret1 : xbsIndex_r4/Reinterpret  force_arith_type=on  arith_type="Signed  (2's comp)"  force_bin_pt=on  bin_pt=0  block_type=reinterpret
  Reinterpret2 : xbsIndex_r4/Reinterpret  force_arith_type=on  arith_type="Signed  (2's comp)"  force_bin_pt=on  bin_pt=0  block_type=reinterpret
  Slice1 : xbsIndex_r4/Slice  nbits=30  boolean_output=off  mode=Lower Bit Location + Width  bit1=0  base1=MSB of Input  bit0=18  base0=LSB of Input  dbl_ovrd=off  block_type=slice
  Slice3 : xbsIndex_r4/Slice  nbits=18  boolean_output=off  mode=Lower Bit Location + Width  bit1=0  base1=MSB of Input  bit0=0  base0=LSB of Input  dbl_ovrd=off  block_type=slice
  A : Outport
  B : Outport  Port=2
  wires:
  A:B/1 -> Slice3/1, Slice1/1
  Slice3/1 -> Reinterpret1/1  "Slice3_out1"
  Slice1/1 -> Reinterpret2/1  "Slice1_out1"
  Reinterpret2/1 -> A/1
  Reinterpret1/1 -> B/1

== system kurtosis_single_channel_subblocks/kurtosis_acc_bank/abs_x_sq_acc/cram ==
  In1 : Inport
  In2 : Inport  Port=2
  Concat : xbsIndex_r4/Concat  num_inputs=2  dbl_ovrd=off  block_type=concat
  Reinterp1 : xbsIndex_r4/Reinterpret  force_arith_type=on  arith_type=Unsigned  force_bin_pt=on  bin_pt=0  block_type=reinterpret
  Reinterp2 : xbsIndex_r4/Reinterpret  force_arith_type=on  arith_type=Unsigned  force_bin_pt=on  bin_pt=0  block_type=reinterpret
  Out : Outport
  wires:
  Concat/1 -> Out/1
  Reinterp2/1 -> Concat/2
  Reinterp1/1 -> Concat/1
  In2/1 -> Reinterp2/1
  In1/1 -> Reinterp1/1

== system kurtosis_single_channel_subblocks/kurtosis_acc_bank/abs_x_sq_acc/dsp48e_ctrl_init_xblock12 ==
  alumode0 : xbsIndex_r4/Constant  const=0  gui_display_data_type=Fixed-point  arith_type=Unsigned  n_bits=4  bin_pt=0  preci_type=Single  exp_width=8  frac_width=24  explicit_period=off  period=1  equ=P=C  opselect=C  inp2=PCIN>>17  opr=+  inp1=P  carry=CIN  dbl_ovrd=off  block_type=constant
  carryin0 : xbsIndex_r4/Constant  const=0  gui_display_data_type=Fixed-point  arith_type=Unsigned  n_bits=1  bin_pt=0  preci_type=Single  exp_width=8  frac_width=24  explicit_period=off  period=1  equ=P=C  opselect=C  inp2=PCIN>>17  opr=+  inp1=P  carry=CIN  dbl_ovrd=off  block_type=constant
  carryinsel0 : xbsIndex_r4/Constant  const=0  gui_display_data_type=Fixed-point  arith_type=Unsigned  n_bits=3  bin_pt=0  preci_type=Single  exp_width=8  frac_width=24  explicit_period=off  period=1  equ=P=C  opselect=C  inp2=PCIN>>17  opr=+  inp1=P  carry=CIN  dbl_ovrd=off  block_type=constant
  opmode0 : xbsIndex_r4/Constant  const=44  gui_display_data_type=Fixed-point  arith_type=Unsigned  n_bits=7  bin_pt=0  preci_type=Single  exp_width=8  frac_width=24  explicit_period=off  period=1  equ=P=C  opselect=C  inp2=PCIN>>17  opr=+  inp1=P  carry=CIN  dbl_ovrd=off  block_type=constant
  opmode : Outport
  alumode : Outport  Port=2
  carryin : Outport  Port=3
  carryinsel : Outport  Port=4
  wires:
  opmode0/1 -> opmode/1
  carryinsel0/1 -> carryinsel/1
  carryin0/1 -> carryin/1
  alumode0/1 -> alumode/1

== system kurtosis_single_channel_subblocks/kurtosis_acc_bank/abs_x_sq_acc/dsp48e_ctrl_init_xblock13 ==
  alumode0 : xbsIndex_r4/Constant  const=0  gui_display_data_type=Fixed-point  arith_type=Unsigned  n_bits=4  bin_pt=0  preci_type=Single  exp_width=8  frac_width=24  explicit_period=off  period=1  equ=P=C  opselect=C  inp2=PCIN>>17  opr=+  inp1=P  carry=CIN  dbl_ovrd=off  block_type=constant
  carryin0 : xbsIndex_r4/Constant  const=0  gui_display_data_type=Fixed-point  arith_type=Unsigned  n_bits=1  bin_pt=0  preci_type=Single  exp_width=8  frac_width=24  explicit_period=off  period=1  equ=P=C  opselect=C  inp2=PCIN>>17  opr=+  inp1=P  carry=CIN  dbl_ovrd=off  block_type=constant
  carryinsel0 : xbsIndex_r4/Constant  const=0  gui_display_data_type=Fixed-point  arith_type=Unsigned  n_bits=3  bin_pt=0  preci_type=Single  exp_width=8  frac_width=24  explicit_period=off  period=1  equ=P=C  opselect=C  inp2=PCIN>>17  opr=+  inp1=P  carry=CIN  dbl_ovrd=off  block_type=constant
  opmode0 : xbsIndex_r4/Constant  const=35  gui_display_data_type=Fixed-point  arith_type=Unsigned  n_bits=7  bin_pt=0  preci_type=Single  exp_width=8  frac_width=24  explicit_period=off  period=1  equ=P=C  opselect=C  inp2=PCIN>>17  opr=+  inp1=P  carry=CIN  dbl_ovrd=off  block_type=constant
  opmode : Outport
  alumode : Outport  Port=2
  carryin : Outport  Port=3
  carryinsel : Outport  Port=4
  wires:
  opmode0/1 -> opmode/1
  carryinsel0/1 -> carryinsel/1
  carryin0/1 -> carryin/1
  alumode0/1 -> alumode/1

== system kurtosis_single_channel_subblocks/kurtosis_acc_bank/x_acc/c_to_ri ==
  c : Inport
  force_im : xbsIndex_r4/Reinterpret  force_arith_type=on  arith_type="Signed  (2's comp)"  force_bin_pt=on  bin_pt=17  block_type=reinterpret
  force_re : xbsIndex_r4/Reinterpret  force_arith_type=on  arith_type="Signed  (2's comp)"  force_bin_pt=on  bin_pt=17  block_type=reinterpret
  slice_im : xbsIndex_r4/Slice  nbits=18  boolean_output=off  mode=Lower Bit Location + Width  bit1=0  base1=MSB of Input  bit0=0  base0=LSB of Input  dbl_ovrd=off  block_type=slice
  slice_re : xbsIndex_r4/Slice  nbits=18  boolean_output=off  mode=Upper Bit Location + Width  bit1=0  base1=MSB of Input  bit0=0  base0=LSB of Input  dbl_ovrd=off  block_type=slice
  re : Outport
  im : Outport  Port=2
  wires:
  c/1 -> slice_im/1, slice_re/1
  force_im/1 -> im/1
  slice_im/1 -> force_im/1
  force_re/1 -> re/1
  slice_re/1 -> force_re/1
